simulink subsystem "tireTemp"  (R2022b)
settings: Solver=VariableStepAuto  StartTime=0.0  StopTime=10.0  RelTol=1e-3
libraries: tireTemp_lib x12
settings Model: Creator=serga  LastModifiedBy=serga

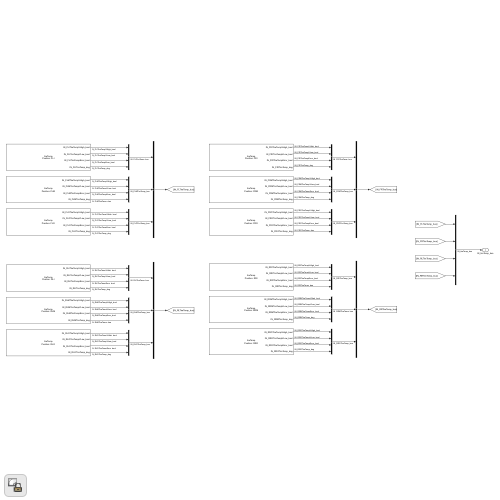
[thumbnail: Simulink's stored preview of the top-level diagram]
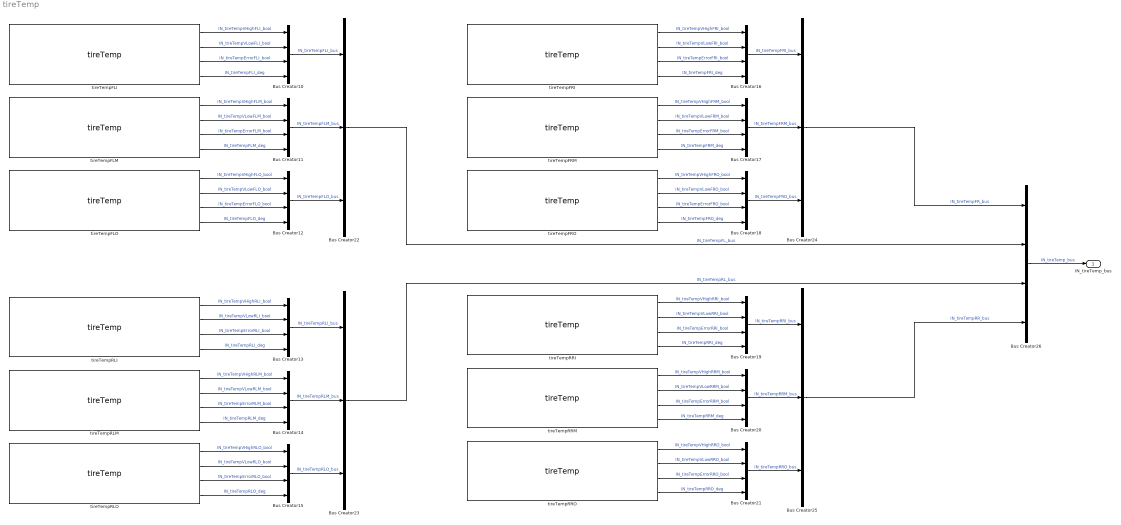
== system tireTemp ==
  Bus Creator{10..21,26} (13 alike) : BusCreator  Inputs=4
  Bus Creator{22..25} (4 alike) : BusCreator  Inputs=3
  tireTempFLI : tireTemp_lib/tireTemp  pos='FLI'
  tireTempFLM : tireTemp_lib/tireTemp  pos='FLM'
  tireTempFLO : tireTemp_lib/tireTemp  pos='FLO'
  tireTempFRI : tireTemp_lib/tireTemp  pos='FRI'
  tireTempFRM : tireTemp_lib/tireTemp  pos='FRM'
  tireTempFRO : tireTemp_lib/tireTemp  pos='FRO'
  tireTempRLI : tireTemp_lib/tireTemp  pos='RLI'
  tireTempRLM : tireTemp_lib/tireTemp  pos='RLM'
  tireTempRLO : tireTemp_lib/tireTemp  pos='RLO'
  tireTempRRI : tireTemp_lib/tireTemp  pos='RRI'
  tireTempRRM : tireTemp_lib/tireTemp  pos='RRM'
  tireTempRRO : tireTemp_lib/tireTemp  pos='RRO'
  IN_tireTemp_bus : Outport
  wires:
  tireTempRLM/3 -> Bus Creator14/3  "IN_tireTempErrorRLM_bool"
  tireTempFLM/4 -> Bus Creator11/4  "IN_tireTempFLM_deg"
  Bus Creator13/1 -> Bus Creator23/1  "IN_tireTempRLI_bus"
  Bus Creator12/1 -> Bus Creator22/3  "IN_tireTempFLO_bus"
  tireTempRRI/1 -> Bus Creator19/1  "IN_tireTempVHighRRI_bool"
  tireTempRRI/4 -> Bus Creator19/4  "IN_tireTempRRI_deg"
  tireTempFRM/3 -> Bus Creator17/3  "IN_tireTempErrorFRM_bool"
  tireTempRLO/1 -> Bus Creator15/1  "IN_tireTempVHighRLO_bool"
  tireTempRRO/1 -> Bus Creator21/1  "IN_tireTempVHighRRO_bool"
  tireTempRRI/3 -> Bus Creator19/3  "IN_tireTempErrorRRI_bool"
  Bus Creator20/1 -> Bus Creator25/2  "IN_tireTempRRM_bus"
  Bus Creator14/1 -> Bus Creator23/2  "IN_tireTempRLM_bus"
  tireTempFRO/3 -> Bus Creator18/3  "IN_tireTempErrorFRO_bool"
  Bus Creator25/1 -> Bus Creator26/4  "IN_tireTempRR_bus"
  Bus Creator23/1 -> Bus Creator26/3  "IN_tireTempRL_bus"
  Bus Creator19/1 -> Bus Creator25/1  "IN_tireTempRRI_bus"
  tireTempFRO/4 -> Bus Creator18/4  "IN_tireTempFRO_deg"
  tireTempRRM/1 -> Bus Creator20/1  "IN_tireTempVHighRRM_bool"
  Bus Creator22/1 -> Bus Creator26/2  "IN_tireTempFL_bus"
  Bus Creator17/1 -> Bus Creator24/2  "IN_tireTempFRM_bus"
  Bus Creator15/1 -> Bus Creator23/3  "IN_tireTempRLO_bus"
  tireTempFLI/3 -> Bus Creator10/3  "IN_tireTempErrorFLI_bool"
  Bus Creator18/1 -> Bus Creator24/3  "IN_tireTempFRO_bus"
  tireTempFLM/3 -> Bus Creator11/3  "IN_tireTempErrorFLM_bool"
  Bus Creator16/1 -> Bus Creator24/1  "IN_tireTempFRI_bus"
  Bus Creator24/1 -> Bus Creator26/1  "IN_tireTempFR_bus"
  tireTempRRM/4 -> Bus Creator20/4  "IN_tireTempRRM_deg"
  tireTempRRM/2 -> Bus Creator20/2  "IN_tireTempVLowRRM_bool"
  tireTempRLI/4 -> Bus Creator13/4  "IN_tireTempRLI_deg"
  Bus Creator21/1 -> Bus Creator25/3  "IN_tireTempRRO_bus"
  Bus Creator10/1 -> Bus Creator22/1  "IN_tireTempFLI_bus"
  tireTempRRO/4 -> Bus Creator21/4  "IN_tireTempRRO_deg"
  tireTempFRI/3 -> Bus Creator16/3  "IN_tireTempErrorFRI_bool"
  tireTempFRO/1 -> Bus Creator18/1  "IN_tireTempVHighFRO_bool"
  tireTempRLI/2 -> Bus Creator13/2  "IN_tireTempVLowRLI_bool"
  tireTempRRI/2 -> Bus Creator19/2  "IN_tireTempVLowRRI_bool"
  tireTempFLO/4 -> Bus Creator12/4  "IN_tireTempFLO_deg"
  tireTempFLO/3 -> Bus Creator12/3  "IN_tireTempErrorFLO_bool"
  tireTempFRM/2 -> Bus Creator17/2  "IN_tireTempVLowFRM_bool"
  tireTempFLO/2 -> Bus Creator12/2  "IN_tireTempVLowFLO_bool"
  tireTempFLI/4 -> Bus Creator10/4  "IN_tireTempFLI_deg"
  tireTempFLM/2 -> Bus Creator11/2  "IN_tireTempVLowFLM_bool"
  tireTempFLM/1 -> Bus Creator11/1  "IN_tireTempVHighFLM_bool"
  tireTempRLM/1 -> Bus Creator14/1  "IN_tireTempVHighRLM_bool"
  tireTempFLI/1 -> Bus Creator10/1  "IN_tireTempVHighFLI_bool"
  tireTempFRI/4 -> Bus Creator16/4  "IN_tireTempFRI_deg"
  tireTempFRI/2 -> Bus Creator16/2  "IN_tireTempVLowFRI_bool"
  tireTempRRO/2 -> Bus Creator21/2  "IN_tireTempVLowRRO_bool"
  tireTempFLO/1 -> Bus Creator12/1  "IN_tireTempVHighFLO_bool"
  tireTempRRM/3 -> Bus Creator20/3  "IN_tireTempErrorRRM_bool"
  tireTempRLM/4 -> Bus Creator14/4  "IN_tireTempRLM_deg"
  tireTempFRO/2 -> Bus Creator18/2  "IN_tireTempVLowFRO_bool"
  tireTempFRM/1 -> Bus Creator17/1  "IN_tireTempVHighFRM_bool"
  tireTempFRM/4 -> Bus Creator17/4  "IN_tireTempFRM_deg"
  Bus Creator11/1 -> Bus Creator22/2  "IN_tireTempFLM_bus"
  tireTempFLI/2 -> Bus Creator10/2  "IN_tireTempVLowFLI_bool"
  tireTempRLO/3 -> Bus Creator15/3  "IN_tireTempErrorRLO_bool"
  tireTempRLO/2 -> Bus Creator15/2  "IN_tireTempVLowRLO_bool"
  tireTempRLI/1 -> Bus Creator13/1  "IN_tireTempVHighRLI_bool"
  tireTempRRO/3 -> Bus Creator21/3  "IN_tireTempErrorRRO_bool"
  tireTempFRI/1 -> Bus Creator16/1  "IN_tireTempVHighFRI_bool"
  tireTempRLO/4 -> Bus Creator15/4  "IN_tireTempRLO_deg"
  tireTempRLM/2 -> Bus Creator14/2  "IN_tireTempVLowRLM_bool"
  tireTempRLI/3 -> Bus Creator13/3  "IN_tireTempErrorRLI_bool"
  Bus Creator26/1 -> IN_tireTemp_bus/1  "IN_tireTemp_bus"
